simulink model "TrajectoryDictionaryGenerator"  (R2019b)
settings: Solver=VariableStepAuto  StartTime=0.0  StopTime=10.0  RelTol=1e-3
settings Model: Creator=loker  LastModifiedBy=loker

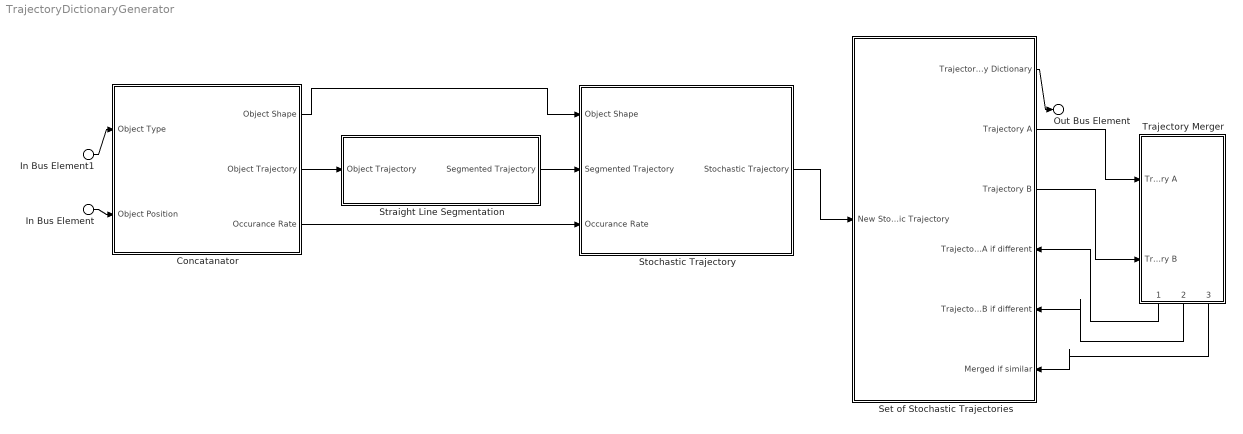
== system TrajectoryDictionaryGenerator ==
  In Bus Element1 : Inport  PortName=Object Type
  In Bus Element : Inport  Port=2  PortName=Object Position
  Concatanator : Subsystem
      settings: PortSchema="{\"entries\":[{\"content\":{\"headerSize\":26,\"margin\":15,\"minimumSpacing\":25,\"sides\":[{\"content\":{\"connectorIds\":[\"In1\",\"In2\"]},\"type\":\"ConnectorPlacement.EquallySpacedRectSide\",\"uuid\":\"e969fe28-f86a-4134-aa48-ac5e7d1e883d\"},{\"content\":{\"connectorIds\":[\"Out1\",\"Out2\",\"Out3\"],\"side\":\"RIGHT\"},\"type\":\"ConnectorPlacement.EquallySpacedRectSide\",\"uuid\":\"60451ad4-053f-474e-b513-91540490c4d6\"},{\"content\":{\"connectorIds\":[],\"side\":\"TOP\"},\"type\":\"ConnectorPlacement.EquallySpacedRectSide\",\"uuid\":\"8c0a71ec-10d4-4c65-a834-1a5cda01dd40\"}]},\"type\":\"ConnectorPlacement.EquallySpacedConnector\",\"uuid\":\"9b9a34e7-bab3-4005-850a-799bc8dbb258\"}],\"packageUris\":[\"http://schema.mathworks.com/mf0/Connector/19700101\"],\"version\":\"1.0\"}"
  Set of Stochastic Trajectories : Subsystem
      settings: PortSchema="{\"entries\":[{\"content\":{\"headerSize\":26,\"margin\":15,\"minimumSpacing\":25,\"sides\":[{\"content\":{\"connectorIds\":[\"In4\"]},\"type\":\"ConnectorPlacement.EquallySpacedRectSide\",\"uuid\":\"e969fe28-f86a-4134-aa48-ac5e7d1e883d\"},{\"content\":{\"connectorIds\":[\"Out1\",\"Out2\",\"Out3\",\"In1\",\"In2\",\"In3\"],\"side\":\"RIGHT\"},\"type\":\"ConnectorPlacement.EquallySpacedRectSide\",\"uuid\":\"60451ad4-053f-474e-b513-91540490c4d6\"},{\"content\":{\"connectorIds\":[],\"side\":\"TOP\"},\"type\":\"ConnectorPlacement.EquallySpacedRectSide\",\"uuid\":\"8c0a71ec-10d4-4c65-a834-1a5cda01dd40\"}]},\"type\":\"ConnectorPlacement.EquallySpacedConnector\",\"uuid\":\"9b9a34e7-bab3-4005-850a-799bc8dbb258\"}],\"packageUris\":[\"http://schema.mathworks.com/mf0/Connector/19700101\"],\"version\":\"1.0\"}"
  Stochastic Trajectory : Subsystem
      settings: PortSchema="{\"entries\":[{\"content\":{\"headerSize\":26,\"margin\":15,\"minimumSpacing\":25,\"sides\":[{\"content\":{\"connectorIds\":[\"In1\",\"In2\",\"In3\"]},\"type\":\"ConnectorPlacement.EquallySpacedRectSide\",\"uuid\":\"e969fe28-f86a-4134-aa48-ac5e7d1e883d\"},{\"content\":{\"connectorIds\":[\"Out1\"],\"side\":\"RIGHT\"},\"type\":\"ConnectorPlacement.EquallySpacedRectSide\",\"uuid\":\"60451ad4-053f-474e-b513-91540490c4d6\"},{\"content\":{\"connectorIds\":[],\"side\":\"TOP\"},\"type\":\"ConnectorPlacement.EquallySpacedRectSide\",\"uuid\":\"8c0a71ec-10d4-4c65-a834-1a5cda01dd40\"}]},\"type\":\"ConnectorPlacement.EquallySpacedConnector\",\"uuid\":\"9b9a34e7-bab3-4005-850a-799bc8dbb258\"}],\"packageUris\":[\"http://schema.mathworks.com/mf0/Connector/19700101\"],\"version\":\"1.0\"}"
  Straight Line Segmentation : Subsystem
      settings: PortSchema="{\"entries\":[{\"content\":{\"headerSize\":26,\"margin\":15,\"minimumSpacing\":25,\"sides\":[{\"content\":{\"connectorIds\":[\"In1\"]},\"type\":\"ConnectorPlacement.EquallySpacedRectSide\",\"uuid\":\"e969fe28-f86a-4134-aa48-ac5e7d1e883d\"},{\"content\":{\"connectorIds\":[\"Out1\"],\"side\":\"RIGHT\"},\"type\":\"ConnectorPlacement.EquallySpacedRectSide\",\"uuid\":\"60451ad4-053f-474e-b513-91540490c4d6\"},{\"content\":{\"connectorIds\":[],\"side\":\"TOP\"},\"type\":\"ConnectorPlacement.EquallySpacedRectSide\",\"uuid\":\"8c0a71ec-10d4-4c65-a834-1a5cda01dd40\"}]},\"type\":\"ConnectorPlacement.EquallySpacedConnector\",\"uuid\":\"9b9a34e7-bab3-4005-850a-799bc8dbb258\"}],\"packageUris\":[\"http://schema.mathworks.com/mf0/Connector/19700101\"],\"version\":\"1.0\"}"
  Trajectory Merger : Subsystem
      settings: PortSchema="{\"entries\":[{\"content\":{\"headerSize\":26,\"margin\":15,\"minimumSpacing\":25,\"sides\":[{\"content\":{\"connectorIds\":[\"In1\",\"In2\"]},\"type\":\"ConnectorPlacement.EquallySpacedRectSide\",\"uuid\":\"e969fe28-f86a-4134-aa48-ac5e7d1e883d\"},{\"content\":{\"connectorIds\":[],\"side\":\"RIGHT\"},\"type\":\"ConnectorPlacement.EquallySpacedRectSide\",\"uuid\":\"60451ad4-053f-474e-b513-91540490c4d6\"},{\"content\":{\"connectorIds\":[],\"side\":\"TOP\"},\"type\":\"ConnectorPlacement.EquallySpacedRectSide\",\"uuid\":\"8c0a71ec-10d4-4c65-a834-1a5cda01dd40\"},{\"content\":{\"connectorIds\":[\"Out1\",\"Out2\",\"Out3\"],\"side\":\"BOTTOM\"},\"type\":\"ConnectorPlacement.EquallySpacedRectSide\",\"uuid\":\"02c689ff-4ba3-4f96-99a3-ab0ff69e93fe\"}]},\"type\":\"ConnectorPlacement.EquallySpacedConnector\",\"uuid\":\"9b9a34e7-bab3-4005-850a-799bc8dbb258\"}],\"packageUris\":[\"http://schema.mathworks.com/mf0/Connector/19700101\"],\"version\":\"1.0\"}"
  Out Bus Element : Outport  PortName=Trajectory Dictionary
  wires:
  In Bus Element/1 -> Concatanator/2(Object Position)
  Concatanator/2(Object Trajectory) -> Straight Line Segmentation/1(Object Trajectory)
  Straight Line Segmentation/1(Segmented Trajectory) -> Stochastic Trajectory/2(Segmented Trajectory)
  Stochastic Trajectory/1(Stochastic Trajectory) -> Set of Stochastic Trajectories/4(" New Stochastic Trajectory")
  Set of Stochastic Trajectories/2(Trajectory A) -> Trajectory Merger/1(Trajectory A)
  Set of Stochastic Trajectories/3(Trajectory B) -> Trajectory Merger/2(Trajectory B)
  Trajectory Merger/1(Trajecteory A if different) -> Set of Stochastic Trajectories/1(Trajectory A if different)
  Trajectory Merger/2(Trajectory B if different) -> Set of Stochastic Trajectories/2(Trajectory B if different)
  Trajectory Merger/3(Merged if similar) -> Set of Stochastic Trajectories/3(Merged if similar)
  Set of Stochastic Trajectories/1(Trajectory Dictionary) -> Out Bus Element/1
  Concatanator/1(Object Shape) -> Stochastic Trajectory/1(Object Shape)
  Concatanator/3(Occurance Rate) -> Stochastic Trajectory/3(Occurance Rate)
  In Bus Element1/1 -> Concatanator/1(Object Type)

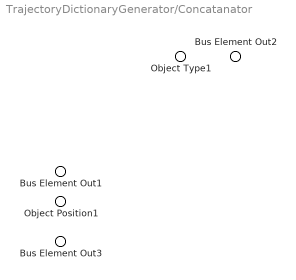
== system TrajectoryDictionaryGenerator/Concatanator ==
  Object Type1 : Inport  PortName=Object Type
  Object Position1 : Inport  Port=2  PortName=Object Position
  Bus Element Out2 : Outport  PortName=Object Shape
  Bus Element Out1 : Outport  Port=2  PortName=Object Trajectory
  Bus Element Out3 : Outport  Port=3  PortName=Occurance Rate

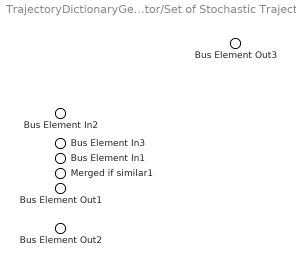
== system TrajectoryDictionaryGenerator/Set of Stochastic Trajectories ==
  Bus Element In2 : Inport  PortName=Trajectory A if different
  Bus Element In3 : Inport  Port=2  PortName=Trajectory B if different
  Merged if similar1 : Inport  Port=3  PortName=Merged if similar
  Bus Element In1 : Inport  Port=4  PortName=New Stochastic Trajectory
  Bus Element Out3 : Outport  PortName=Trajectory Dictionary
  Bus Element Out1 : Outport  Port=2  PortName=Trajectory A
  Bus Element Out2 : Outport  Port=3  PortName=Trajectory B

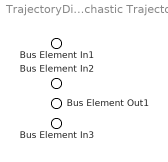
== system TrajectoryDictionaryGenerator/Stochastic Trajectory ==
  Bus Element In1 : Inport  PortName=Object Shape
  Bus Element In2 : Inport  Port=2  PortName=Segmented Trajectory
  Bus Element In3 : Inport  Port=3  PortName=Occurance Rate
  Bus Element Out1 : Outport  PortName=Stochastic Trajectory

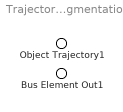
== system TrajectoryDictionaryGenerator/Straight Line Segmentation ==
  Object Trajectory1 : Inport  PortName=Object Trajectory
  Bus Element Out1 : Outport  PortName=Segmented Trajectory

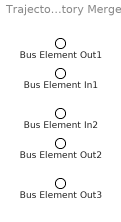
== system TrajectoryDictionaryGenerator/Trajectory Merger ==
  Bus Element In1 : Inport  PortName=Trajectory A
  Bus Element In2 : Inport  Port=2  PortName=Trajectory B
  Bus Element Out1 : Outport  PortName=Trajecteory A if different
  Bus Element Out2 : Outport  Port=2  PortName=Trajectory B if different
  Bus Element Out3 : Outport  Port=3  PortName=Merged if similar
